simulink model "Planar_Full_NL_Subsystems_GroupParameters"  (R2016a)
settings: Solver=VariableStepAuto  StartTime=0.0  StopTime=10.0  RelTol=1e-3
values from neighbouring files (symbols this model uses):
  k_reg = 6.09    [Systemdesign_XY.m]
  k_s = double(subs(k_s,T_z,1))    [Systemdesign_XY.m]
  T_1 = T_sampl/2    (= 0.0035)    [Systemdesign_XY.m]
  T_r = T_1*0.5    (= 0.00175)    [Systemdesign_XY.m]
  T_x_AP = 0    [Computation.m]    (also in Computation_with_Langrange.m)
  T_y_AP = 0    [Computation.m]    (also in Computation_with_Langrange.m)
  T_z_AP = 0    [Computation.m]    (also in Computation_with_Langrange.m)
  x_AP = [0;0;0;0]    [Computation.m]    (also in Computation_with_Langrange.m = [0 0 0 0])
undefined symbols (not defined in the file or in its folder): alpha, beta, K_xz, K_yz
libraries: simulink x3
settings Model: Creator=Florian  LastModifiedBy=Florian

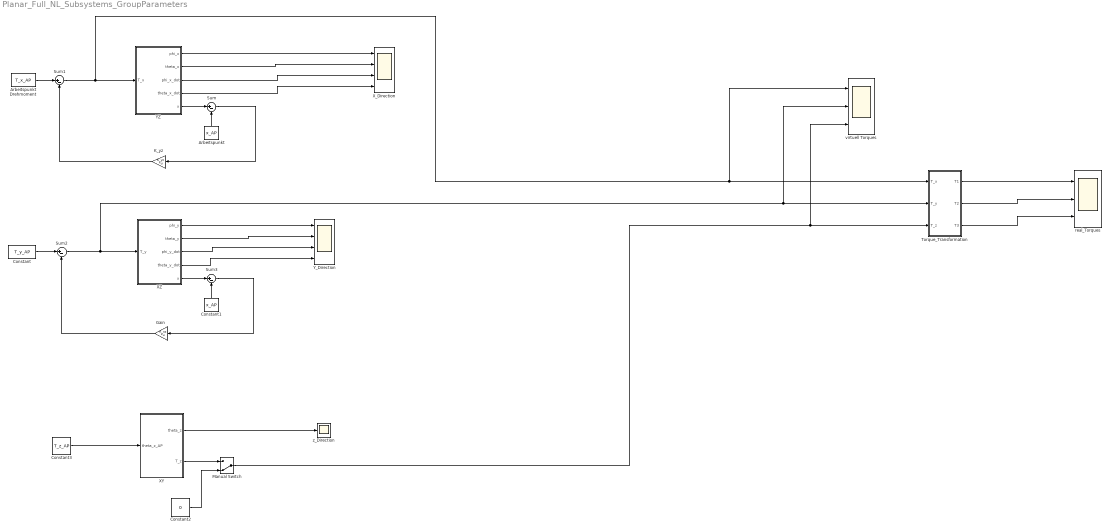
== system Planar_Full_NL_Subsystems_GroupParameters ==
  Arbeitspunkt : Constant  Value=x_AP
  Arbeitspunkt Drehmoment : Constant  Value=T_x_AP
  Constant : Constant  Value=T_y_AP
  Constant1 : Constant  Value=x_AP
  Constant2 : Constant  Value=0
  Constant3 : Constant  Value=T_z_AP
  Gain : Gain  Gain=K_xz  Multiplication=Matrix(K*u) (u vector)
  K_yz : Gain  Gain=K_yz  Multiplication=Matrix(K*u) (u vector)
  Manual Switch : ManualSwitch  CurrentSetting=0
  Sum{,1..3} (4 alike) : Sum  Inputs=|+-
  Torque_Transformation : Subsystem
  XY : Subsystem
  XZ : Subsystem
  X_Direction : Scope  NumInputPorts=4
  YZ : Subsystem
  Y_Direction : Scope  NumInputPorts=4
  real_Torques : Scope  NumInputPorts=3
  virtuell Torques : Scope  NumInputPorts=3
  z_Direction : Scope
  wires:
  K_yz/1 -> Sum1/2
  Arbeitspunkt Drehmoment/1 -> Sum1/1
  Arbeitspunkt/1 -> Sum/2
  Sum/1 -> K_yz/1
  Constant1/1 -> Sum3/2
  Constant/1 -> Sum2/1
  Gain/1 -> Sum2/2
  Constant3/1 -> XY/1("theta_z_AP ")
  Sum3/1 -> Gain/1
  Sum1/1 -> virtuell Torques/1, Torque_Transformation/1(T_x), YZ/1("T_x ")
  YZ/5(x) -> Sum/1
  Sum2/1 -> virtuell Torques/2, Torque_Transformation/2(T_y), XZ/1("T_y ")
  XZ/5(x) -> Sum3/1
  YZ/1(phi_x) -> X_Direction/1
  YZ/2(theta_x) -> X_Direction/2
  YZ/3(phi_x_dot) -> X_Direction/3
  YZ/4(theta_x_dot) -> X_Direction/4
  XZ/1(phi_y) -> Y_Direction/1
  XZ/2(theta_y) -> Y_Direction/2
  XZ/3(phi_y_dot) -> Y_Direction/3
  XZ/4(theta_y_dot) -> Y_Direction/4
  XY/1("theta_z ") -> z_Direction/1
  Torque_Transformation/1(T1) -> real_Torques/1
  Torque_Transformation/2(T2) -> real_Torques/2
  Torque_Transformation/3(T3) -> real_Torques/3
  XY/2(T_z) -> Manual Switch/1
  Manual Switch/1 -> virtuell Torques/3, Torque_Transformation/3(T_z)
  Constant2/1 -> Manual Switch/2

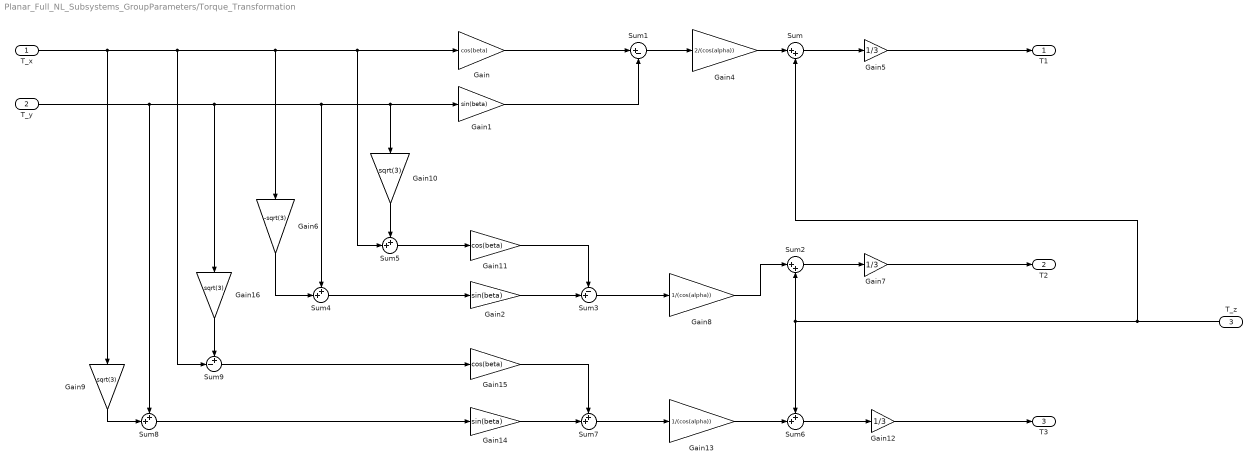
== system Planar_Full_NL_Subsystems_GroupParameters/Torque_Transformation ==
  T_x : Inport
  T_y : Inport  Port=2
  T_z : Inport  Port=3
  Gain : Gain  Gain=cos(beta)
  Gain1 : Gain  Gain=sin(beta)
  Gain10 : Gain  Gain=sqrt(3)
  Gain11 : Gain  Gain=cos(beta)
  Gain12 : Gain  Gain=1/3
  Gain13 : Gain  Gain=1/(cos(alpha))
  Gain14 : Gain  Gain=sin(beta)
  Gain15 : Gain  Gain=cos(beta)
  Gain16 : Gain  Gain=sqrt(3)
  Gain2 : Gain  Gain=sin(beta)
  Gain4 : Gain  Gain=2/(cos(alpha))
  Gain5 : Gain  Gain=1/3
  Gain6 : Gain  Gain=-sqrt(3)
  Gain7 : Gain  Gain=1/3
  Gain8 : Gain  Gain=1/(cos(alpha))
  Gain9 : Gain  Gain=sqrt(3)
  Sum : Sum  Inputs=|++
  Sum1 : Sum  Inputs=|+-
  Sum2 : Sum  Inputs=|++
  Sum3 : Sum  Inputs=-+|
  Sum{4..8} (5 alike) : Sum  Inputs=++|
  Sum9 : Sum  Inputs=+-|
  T1 : Outport
  T2 : Outport  Port=2
  T3 : Outport  Port=3
  wires:
  Sum1/1 -> Gain4/1
  Sum/1 -> Gain5/1
  Gain5/1 -> T1/1
  Sum3/1 -> Gain8/1
  Sum8/1 -> Gain14/1
  Sum2/1 -> Gain7/1
  Gain11/1 -> Sum3/1
  Sum4/1 -> Gain2/1
  T_x/1 -> Sum9/2, Gain/1, Sum5/2, Gain6/1, Gain9/1
  Gain10/1 -> Sum5/1
  Gain12/1 -> T3/1
  Gain8/1 -> Sum2/1
  T_z/1 -> Sum2/2, Sum6/1, Sum/2
  Gain2/1 -> Sum3/2
  Gain1/1 -> Sum1/2
  T_y/1 -> Gain16/1, Gain1/1, Gain10/1, Sum4/1, Sum8/1
  Gain6/1 -> Sum4/2
  Sum5/1 -> Gain11/1
  Gain7/1 -> T2/1
  Gain4/1 -> Sum/1
  Gain13/1 -> Sum6/2
  Sum7/1 -> Gain13/1
  Gain/1 -> Sum1/1
  Sum6/1 -> Gain12/1
  Gain9/1 -> Sum8/2
  Sum9/1 -> Gain15/1
  Gain16/1 -> Sum9/1
  Gain15/1 -> Sum7/1
  Gain14/1 -> Sum7/2

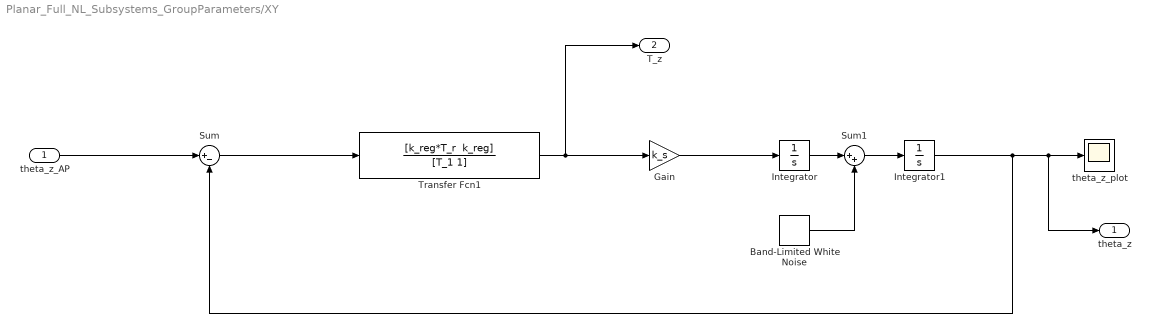
== system Planar_Full_NL_Subsystems_GroupParameters/XY ==
  "theta_z_AP " : Inport
  Band-Limited White Noise : simulink/Sources/Band-Limited White Noise  Cov=[0.1^2]  Ts=1/92  seed=[23341]
  Gain : Gain  Gain=k_s
  Integrator : Integrator
  Integrator1 : Integrator  InitialCondition=pi/32
  Sum : Sum  Inputs=|+-
  Sum1 : Sum  Inputs=|++
  Transfer Fcn1 : TransferFcn  Numerator="[k_reg*T_r  k_reg]"  Denominator=[T_1 1]
  theta_z_plot : Scope
  "theta_z " : Outport
  T_z : Outport  Port=2
  wires:
  "theta_z_AP "/1 -> Sum/1
  Transfer Fcn1/1 -> T_z/1, Gain/1
  Band-Limited White Noise/1 -> Sum1/2
  Gain/1 -> Integrator/1
  Integrator1/1 -> "theta_z "/1, theta_z_plot/1, Sum/2
  Sum/1 -> Transfer Fcn1/1
  Sum1/1 -> Integrator1/1
  Integrator/1 -> Sum1/1

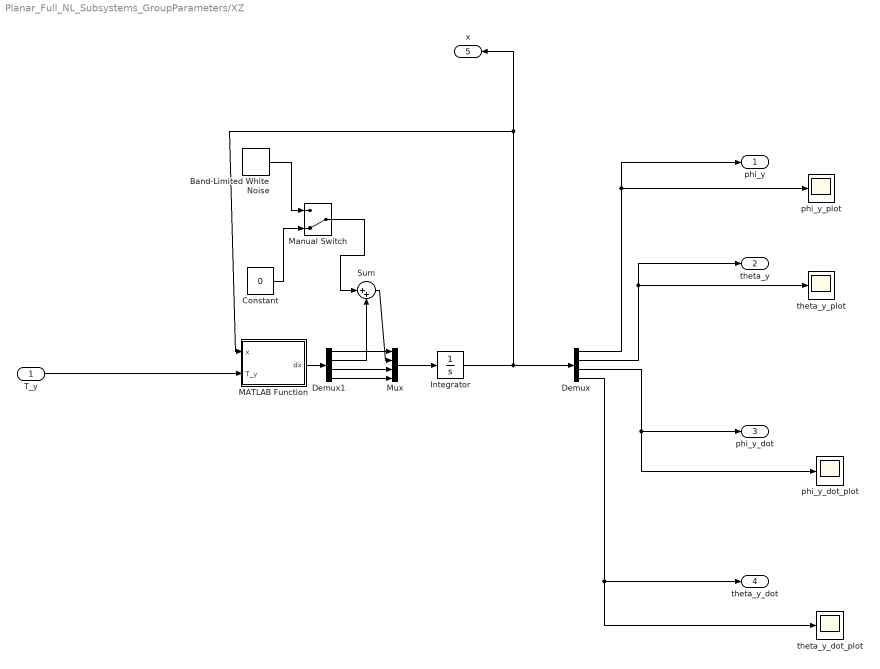
== system Planar_Full_NL_Subsystems_GroupParameters/XZ ==
  "T_y " : Inport
  Band-Limited White Noise : simulink/Sources/Band-Limited White Noise  Cov=[0.1^2]  Ts=1/92  seed=[23341]
  Constant : Constant  Value=0
  Demux : Demux
  Demux1 : Demux
  Integrator : Integrator  InitialCondition=[0 pi/32 0 0]
  MATLAB Function : MATLAB Function  TreatAsAtomicUnit=on
  Manual Switch : ManualSwitch  CurrentSetting=0
  Mux : Mux
  Sum : Sum  Inputs=|++
  phi_y_dot_plot : Scope
  phi_y_plot : Scope
  theta_y_dot_plot : Scope
  theta_y_plot : Scope
  phi_y : Outport
  theta_y : Outport  Port=2
  phi_y_dot : Outport  Port=3
  theta_y_dot : Outport  Port=4
  x : Outport  Port=5
  wires:
  Integrator/1 -> x/1, MATLAB Function/1(x), Demux/1
  Demux/4 -> theta_y_dot/1, theta_y_dot_plot/1
  Demux/1 -> phi_y/1, phi_y_plot/1
  "T_y "/1 -> MATLAB Function/2(T_y)
  MATLAB Function/1(dx) -> Demux1/1
  Demux1/4 -> Mux/4
  Demux1/3 -> Mux/3
  Sum/1 -> Mux/2
  Mux/1 -> Integrator/1
  Demux1/2 -> Sum/2
  Demux1/1 -> Mux/1
  Demux/3 -> phi_y_dot/1, phi_y_dot_plot/1
  Demux/2 -> theta_y/1, theta_y_plot/1
  Manual Switch/1 -> Sum/1
  Constant/1 -> Manual Switch/2
  Band-Limited White Noise/1 -> Manual Switch/1

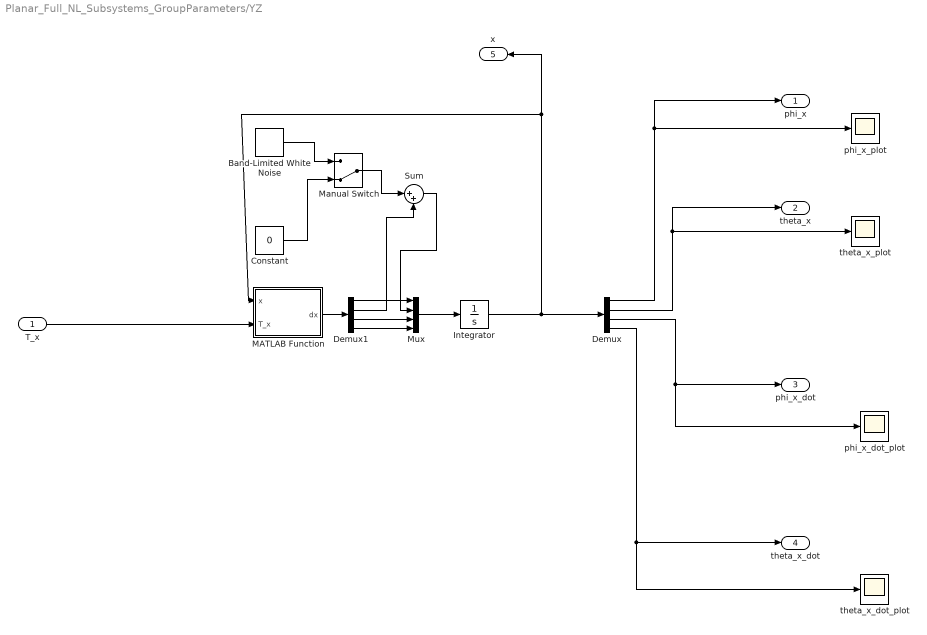
== system Planar_Full_NL_Subsystems_GroupParameters/YZ ==
  "T_x " : Inport
  Band-Limited White Noise : simulink/Sources/Band-Limited White Noise  Cov=[0.1^2]  Ts=1/92  seed=[23341]
  Constant : Constant  Value=0
  Demux : Demux
  Demux1 : Demux
  Integrator : Integrator  InitialCondition=[0 0 0 0]
  MATLAB Function : MATLAB Function  TreatAsAtomicUnit=on
  Manual Switch : ManualSwitch  CurrentSetting=0
  Mux : Mux
  Sum : Sum  Inputs=|++
  phi_x_dot_plot : Scope
  phi_x_plot : Scope
  theta_x_dot_plot : Scope
  theta_x_plot : Scope
  phi_x : Outport
  theta_x : Outport  Port=2
  phi_x_dot : Outport  Port=3
  theta_x_dot : Outport  Port=4
  x : Outport  Port=5
  wires:
  Integrator/1 -> x/1, MATLAB Function/1(x), Demux/1
  Demux/1 -> phi_x/1, phi_x_plot/1
  Demux/2 -> theta_x/1, theta_x_plot/1
  MATLAB Function/1(dx) -> Demux1/1
  Demux/3 -> phi_x_dot/1, phi_x_dot_plot/1
  Demux1/2 -> Sum/2
  Demux1/3 -> Mux/3
  Demux1/1 -> Mux/1
  Sum/1 -> Mux/2
  Mux/1 -> Integrator/1
  "T_x "/1 -> MATLAB Function/2(T_x)
  Demux/4 -> theta_x_dot/1, theta_x_dot_plot/1
  Demux1/4 -> Mux/4
  Manual Switch/1 -> Sum/1
  Band-Limited White Noise/1 -> Manual Switch/1
  Constant/1 -> Manual Switch/2

== matlab function Planar_Full_NL_Subsystems_GroupParameters/XZ/MATLAB Function ==
  data: x input; T_y input; dx output
function dx = fcn_xz(x,T_y)

%Zuweisung Koordinaten und Ableitungen
phi_y =x(1);
theta_y=x(2);
phi_y_dot=x(3);
theta_y_dot=x(4);

phi_y_dotdot = (1125899906842624*(3806346554041953561750000*sin(theta_y)*theta_y_dot^2 + 305940331326383437500000000*T_y + 53252631242683345333265625*sin(theta_y) - 44726853734424728391647232*cos(theta_y)*sin(theta_y) + 33092450061918404608000000*T_y*cos(theta_y)))/(3*(325964702984773560838459351891968000000*cos(theta_y) - 136888781387570427621738503649999454208*cos(theta_y)^2 + 1751672718406792998801379845453369140625));

theta_y_dotdot =  -(281474976710656*(22692737802394437500000000*T_y - 243681411007344587809640625*sin(theta_y) - 1737088888650221254500000*theta_y_dot^2*sin(theta_y) + 132369800247673618432000000*T_y*cos(theta_y) + 1458979938329858622357504*theta_y_dot^2*cos(theta_y)*sin(theta_y)))/(3*(325964702984773560838459351891968000000*cos(theta_y) - 136888781387570427621738503649999454208*cos(theta_y)^2 + 1751672718406792998801379845453369140625));

%Zuweisung Ausgang
dx = [phi_y_dot; theta_y_dot; phi_y_dotdot; theta_y_dotdot];
end

== matlab function Planar_Full_NL_Subsystems_GroupParameters/YZ/MATLAB Function ==
  data: x input; T_x input; dx output

function dx = fcn(x,T_x)

%Zuweisung Koordinaten und Ableitungen
phi_x =x(1);
theta_x=x(2);
phi_x_dot=x(3);
theta_x_dot=x(4);

phi_x_dotdot = (1125899906842624*(3806346554041953561750000*sin(theta_x)*theta_x_dot^2 + 305940331326383437500000000*T_x + 53252631242683345333265625*sin(theta_x) - 44726853734424728391647232*cos(theta_x)*sin(theta_x) + 33092450061918404608000000*T_x*cos(theta_x)))/(3*(325964702984773560838459351891968000000*cos(theta_x) - 136888781387570427621738503649999454208*cos(theta_x)^2 + 1751672718406792998801379845453369140625));

theta_x_dotdot = -(281474976710656*(22692737802394437500000000*T_x - 243681411007344587809640625*sin(theta_x) - 1737088888650221254500000*theta_x_dot^2*sin(theta_x) + 132369800247673618432000000*T_x*cos(theta_x) + 1458979938329858622357504*theta_x_dot^2*cos(theta_x)*sin(theta_x)))/(3*(325964702984773560838459351891968000000*cos(theta_x) - 136888781387570427621738503649999454208*cos(theta_x)^2 + 1751672718406792998801379845453369140625));


% phi_x_dotdot = (0.0355556*(1.65925e33*sin(theta_x)*theta_x_dot^2 + 5.804e34*T_x + 1.26585e35*sin(theta_x) - 8.4019e33*cos(theta_x)*sin(theta_x) + 4.60272e33*T_x*cos(theta_x)))/(6.42314e31*cos(theta_x) - 2.13164e30*cos(theta_x)^2 + 1.63981e32);
% 
% theta_x_dotdot = (0.111111*(6.01665e33*T_x + 2.95242e34*sin(theta_x) + 2.89041e32*theta_x_dot^2*sin(theta_x) - 1.47287e33*T_x*cos(theta_x) - 1.91848e31*theta_x_dot^2*cos(theta_x)*sin(theta_x)))/(6.42314e31*cos(theta_x) - 2.13164e30*cos(theta_x)^2 + 1.63981e32);

%Zuweisung Ausgang
dx = [phi_x_dot; theta_x_dot; phi_x_dotdot; theta_x_dotdot];
end
